simulink model "Junctions4Modified_tmp"  (Simulink 8.3)
settings: Solver=ode45  StartTime=0.0  StopTime=10.0  RelTol=1e-3
settings Model: Creator=scaife  LastModifiedBy=bourbouh  CovSFcnEnable=on  ExtModeAutoUpdateStatusClock=off
settings DataIOCC: SignalLoggingName=sigsOut
settings OptimizationCC: InitFltsAndDblsToZero=on
settings DebuggingCC: SaveWithParameterizedLinksMsg=none  SignalResolutionControl=TryResolveAllWithWarning  SolverPrmCheckMsg=none  MultiTaskDSMMsg=warning  MultiTaskCondExecSysMsg=none  FrameProcessingCompatibilityMsg=error  StateNameClashWarn=none  StrictBusMsg=None
settings HardwareCC: TargetUnknown=on
settings SFSimCC: SimParseCustomCode=off
settings GRTTargetCC: TargetFcnLib=ansi_tfl_tmw.mat  ModelReferenceCompliant=off  ParMdlRefBuildCompliant=off  CompOptLevelCompliant=off  ConcurrentExecutionCompliant=off  GeneratePreprocessorConditionals=Use local settings  MatFileLogging=off  MATLABClassNameForMDSCustomization=Simulink.SoftwareTarget.TargetSpecificTriggerConfigurationBase

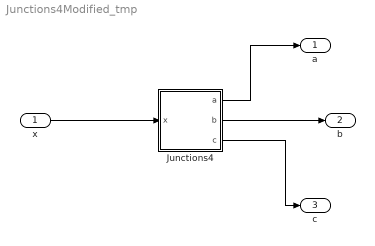
== system Junctions4Modified_tmp ==
  x : Inport
  Junctions4 : Stateflow chart  TreatAsAtomicUnit=on
      settings: PermitHierarchicalResolution=ParametersOnly
  a : Outport
  b : Outport  Port=2
  c : Outport  Port=3
  wires:
  Junctions4/1(a) -> a/1
  Junctions4/2(b) -> b/1
  Junctions4/3(c) -> c/1
  x/1 -> Junctions4/1(x)

== stateflow chart Junctions4 ==
  state TOP
    state A/
      en:c+=1
      ex:c+=10
    state B/
      en:c+=100
      du:c+=1000
    (default) -> A [order 1] : [x<>0]{a+=10}/b+=10
    (default) -> A [order 2] : [x==0]{a+=1}/b+=1
    A -> (junction 6) [order 2] : [x<4]{a+=100}
    A -> (junction 6) [order 1] : [x>=4]{a+=1000}
    (junction 6) -> B [order 1] : [x%%3<>0]
        | {a+=100000}
        | /b+=100000
    (junction 6) -> B [order 2] : [x%%3==0]
        | {a+=10000}
        | /b+=10000
    B -> TOP
  (default) -> TOP
  data: x input int32; a output int32 =111111; b output int32 =111111; c output int32 =111111
